simulink library "Steer_Rack_System"  (R2018b)
settings: Solver=VariableStepAuto  StartTime=0.0  StopTime=10.0  RelTol=1e-3
undefined symbols (not defined in the file): Vehicle
libraries: Steer_Rack x7, sm_car_lib x1
Description:
  | Component of Simscape Vehicle Templates Library
  | 
  | Copyright 2018-2020 The MathWorks, Inc.
settings Model: Creator=smiller  LastModifiedBy=smiller

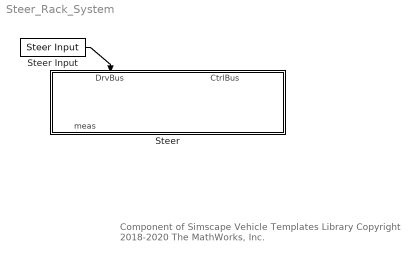
== system Steer_Rack_System ==
  note: Component of Simscape Vehicle Templates Library
      | Copyright 2018-2020 The MathWorks, Inc.
  Steer : Subsystem  Variant=on  VariantControl=Steer  mask{Steer=Vehicle.Chassis.SuspF.Steer, VariantLabel=Vehicle.Chassis.SuspF.Steer.class.Value, InitTriggerDropdown=1}
      mask prompts: Steer "Steer Parameters"; VariantLabel "Variant Label"; InitTriggerDropdown "Initialization Trigger Dropdown"
      mask init:
      | curblk = gcb;
      | 
      | % Set variant for this block 
      | set_param(curblk,'LabelModeActiveChoice',VariantLabel);
      | 
      | % Trigger Mask Initialization for 
      | % variant subsystems below this level
      | sm_car_lib_maskInitTrigger(curblk);
      settings: AttributesFormatString=%<ActiveVariant>
      mask TypeOptions InitTriggerDropdown: 0 | 1
      mask Display: disp(' ');
  Steer Input : sm_car_lib/Inputs/DrvBus/Steer Input  popup_steer_input=Sequence
  wires:
  Steer Input/1 -> Steer/1(DrvBus)

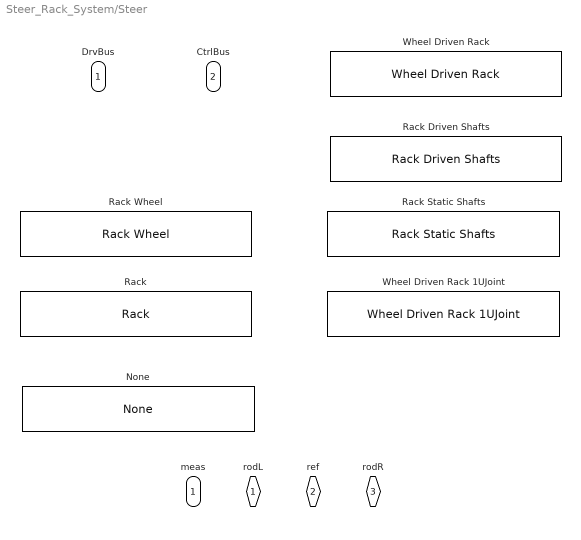
== system Steer_Rack_System/Steer ==
  DrvBus : Inport
  CtrlBus : Inport  Port=2
  None : Steer_Rack/None  SystemSampleTime=-1  VariantControl=None
  Rack : Steer_Rack/Rack  Tag=PublishSubsystem  VariantControl=Rack  hp_mt_rack=Steer.Rack.sMount.Value  hp_out_rack=Steer.Rack.sOutboard.Value  rack_mass=Steer.Rack.m.Value  whl2rack_whlangle=Steer.Ratio_Table.aWheel.Value  whl2rack_rackdisp=Steer.Ratio_Table.xRack.Value  whl2rack_filter=1/Steer.Rack.fActuatorCutoff.Value  clr_rack=Visual.SteeringRack.clr  opc_rack=Visual.part.opc  radius_rack=Visual.SteeringRack.rad  clr_connhp=Visual.hp.clr  opc_connhp=Visual.hp.opc  size_connhp=Visual.hp.rad
  Rack Driven Shafts : Steer_Rack/Rack Driven Shafts  Tag=PublishSubsystem  VariantControl=RackDrivenShafts  InitTriggerDropdown=0  hp_wheel=Steer.Wheel.sMount.Value  wheel_axis_incl=Steer.Wheel.aAxis.Value  hp_mt_rack=Steer.Rack.sMount.Value  hp_out_rack=Steer.Rack.sOutboard.Value  hp_pinion=Steer.Pinion.sMount.Value  len_sha_u=Steer.Shaft_Upper.xLength.Value  sha_u_mass=Steer.Shaft_Upper.m.Value  sha_i_mass=Steer.Shaft_Intermediate.m.Value  len_sha_l=Steer.Shaft_Lower.xLength.Value  sha_l_mass=Steer.Shaft_Lower.m.Value  rad_pinion=Steer.Pinion.xRad.Value  pinion_mass=Steer.Pinion.m.Value  rack_mass=Steer.Rack.m.Value  whl2rack_whlangle=Steer.Ratio_Table.aWheel.Value  whl2rack_rackdisp=Steer.Ratio_Table.xRack.Value  steer_filter=1/Steer.Rack.fActuatorCutoff.Value  clr_rack=Visual.SteeringRack.clr  opc_rack=Visual.part.opc  radius_rack=Visual.SteeringRack.rad  clr_shaft=Visual.SteeringShafts.clr  opc_shaft=Visual.part.opc  size_shaft=Visual.SteeringShafts.rad  clr_pinion=Visual.SteeringPinion.clr  opc_pinion=Visual.part.opc  len_pinion=Visual.SteeringPinion.len  clr_connhp=Visual.hp.clr  opc_connhp=Visual.hp.opc  size_connhp=Visual.hp.rad  clr_wheel=Visual.SteeringWheel.clr  opc_wheel=Visual.part.opc  DriverHuman=Steer.DriverHuman
  Rack Static Shafts : Steer_Rack/Rack Static Shafts  Tag=PublishSubsystem  VariantControl=RackStaticShafts  InitTriggerDropdown=0  hp_wheel=Steer.Wheel.sMount.Value  wheel_axis_incl=Steer.Wheel.aAxis.Value  hp_mt_rack=Steer.Rack.sMount.Value  hp_out_rack=Steer.Rack.sOutboard.Value  hp_pinion=Steer.Pinion.sMount.Value  text_strparts_wheel_m=0  len_sha_u=Steer.Shaft_Upper.xLength.Value  sha_u_mass=Steer.Shaft_Upper.m.Value  sha_i_mass=Steer.Shaft_Intermediate.m.Value  len_sha_l=Steer.Shaft_Lower.xLength.Value  sha_l_mass=Steer.Shaft_Lower.m.Value  rad_pinion=Steer.Pinion.xRad.Value  pinion_mass=Steer.Pinion.m.Value  rack_mass=Steer.Rack.m.Value  whl2rack_whlangle=Steer.Ratio_Table.aWheel.Value  whl2rack_rackdisp=Steer.Ratio_Table.xRack.Value  steer_filter=1/Steer.Rack.fActuatorCutoff.Value  clr_rack=Visual.SteeringRack.clr  opc_rack=Visual.part.opc  radius_rack=Visual.SteeringRack.rad  clr_solid=Visual.SteeringShafts.clr  opc_solid=Visual.part.opc  rad_solid=Visual.SteeringShafts.rad  clr_pinion=Visual.SteeringPinion.clr  opc_pinion=Visual.part.opc  len_pinion=Visual.SteeringPinion.len  clr_connhp=Visual.hp.clr  opc_connhp=Visual.hp.opc  size_connhp=Visual.hp.rad  clr_wheel=Visual.SteeringWheel.clr  opc_wheel=Visual.part.opc  DriverHuman=Steer.DriverHuman
  Rack Wheel : Steer_Rack/Rack Wheel  Tag=PublishSubsystem  VariantControl=RackWheel  InitTriggerDropdown=0  hp_wheel=Steer.Wheel.sMount.Value  wheel_axis_incl=Steer.Wheel.aAxis.Value  hp_mt_rack=Steer.Rack.sMount.Value  hp_out_rack=Steer.Rack.sOutboard.Value  rack_mass=Steer.Rack.m.Value  whl2rack_whlangle=Steer.Ratio_Table.aWheel.Value  whl2rack_rackdisp=Steer.Ratio_Table.xRack.Value  whl2rack_filter=1/Steer.Rack.fActuatorCutoff.Value  clr_rack=Visual.SteeringRack.clr  opc_rack=Visual.part.opc  radius_rack=Visual.SteeringRack.rad  clr_connhp=Visual.hp.clr  opc_connhp=Visual.hp.opc  size_connhp=Visual.hp.rad  clr_wheel=Visual.SteeringWheel.clr  opc_wheel=Visual.part.opc  DriverHuman=Steer.DriverHuman
  Wheel Driven Rack : Steer_Rack/Wheel Driven Rack  Tag=PublishSubsystem  VariantControl=WheelDrivenRack  hp_wheel=Steer.Wheel.sMount.Value  InitTriggerDropdown=0  wheel_axis_incl=Steer.Wheel.aAxis.Value  hp_mt_rack=Steer.Rack.sMount.Value  hp_out_rack=Steer.Rack.sOutboard.Value  hp_pinion=Steer.Pinion.sMount.Value  len_sha_u=Steer.Shaft_Upper.xLength.Value  sha_u_mass=Steer.Shaft_Upper.m.Value  sha_i_mass=Steer.Shaft_Intermediate.m.Value  len_sha_l=Steer.Shaft_Lower.xLength.Value  sha_l_mass=Steer.Shaft_Lower.m.Value  rad_pinion=Steer.Pinion.xRad.Value  pinion_mass=Steer.Pinion.m.Value  rack_mass=Steer.Rack.m.Value  whl2steer_filter=1/Steer.Rack.fActuatorCutoff.Value  clr_rack=Visual.SteeringRack.clr  opc_rack=Visual.part.opc  radius_rack=Visual.SteeringRack.rad  clr_shaft=Visual.SteeringShafts.clr  opc_shaft=Visual.part.opc  size_shaft=Visual.SteeringShafts.rad  clr_pinion=Visual.SteeringPinion.clr  opc_pinion=Visual.part.opc  len_pinion=Visual.SteeringPinion.len  clr_connhp=Visual.hp.clr  opc_connhp=Visual.hp.opc  size_connhp=Visual.hp.rad  clr_wheel=Visual.SteeringWheel.clr  opc_wheel=Visual.part.opc  DriverHuman=Steer.DriverHuman
  Wheel Driven Rack 1UJoint : Steer_Rack/Wheel Driven Rack 1UJoint  Tag=PublishSubsystem  VariantControl=WheelDrivenRack1UJoint  hp_wheel=Steer.Wheel.sMount.Value  InitTriggerDropdown=0  wheel_axis_incl=Steer.Wheel.aAxis.Value  hp_mt_rack=Steer.Rack.sMount.Value  hp_out_rack=Steer.Rack.sOutboard.Value  hp_pinion=Steer.Pinion.sMount.Value  len_sha_u=Steer.Shaft_Upper.xLength.Value  sha_u_mass=Steer.Shaft_Upper.m.Value  sha_l_mass=Steer.Shaft_Lower.m.Value  rad_pinion=Steer.Pinion.xRad.Value  pinion_mass=Steer.Pinion.m.Value  rack_mass=Steer.Rack.m.Value  whl2steer_filter=1/Steer.Rack.fActuatorCutoff.Value  clr_rack=Visual.SteeringRack.clr  opc_rack=Visual.part.opc  radius_rack=Visual.SteeringRack.rad  clr_shaft=Visual.SteeringShafts.clr  opc_shaft=Visual.part.opc  size_shaft=Visual.SteeringShafts.rad  clr_pinion=Visual.SteeringPinion.clr  opc_pinion=Visual.part.opc  len_pinion=Visual.SteeringPinion.len  clr_connhp=Visual.hp.clr  opc_connhp=Visual.hp.opc  size_connhp=Visual.hp.rad  clr_wheel=Visual.SteeringWheel.clr  opc_wheel=Visual.part.opc  DriverHuman=Steer.DriverHuman
  " rodL" : PMIOPort  Side=Right
  " ref" : PMIOPort  Port=2  Side=Right
  " rodR" : PMIOPort  Port=3  Side=Right
  " meas" : Outport
